simulink model "calibration"  (R2020b)
settings: Solver=VariableStepAuto  StartTime=0.0  StopTime=30  RelTol=1e-3
values from neighbouring files (symbols this model uses):
  aubr = -8:0.05:5    [generate_calibration.m]
  tablebr = zeros(length(vubr),length(aubr))    [generate_calibration.m]
  vubr = 0:0.05:50    [generate_calibration.m]
  x = x-0.1    (= -0.1)    [brake_calibration.m]    (also in thr_calibration.m = 0.05)
libraries: Solver_SF x1
settings Model: Creator=wwcong  LastModifiedBy=mepupu
settings DataIOCC: ReturnWorkspaceOutputs=off
settings DebuggingCC: ArithmeticOperatorsInVariantConditions=warning
settings SFSimCC: SimUseLocalCustomCode=off  CustomCodeUndefinedFunction=UseInterfaceOnly
settings RTWCC: RTWUseLocalCustomCode=off

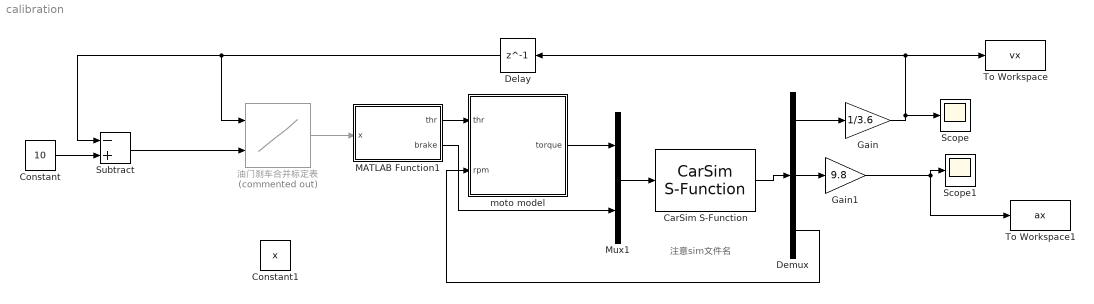
== system calibration ==
  note: 注意sim文件名
  CarSim S-Function : Solver_SF/CarSim S-Function  Priority=1  SIMFILE=simfile.sim
  Constant : Constant  Value=10
  Constant1 : Constant  Value=x
  Delay : Delay  DelayLength=1
  Demux : Demux  Outputs=3
  Gain : Gain  Gain=1/3.6
  Gain1 : Gain  Gain=9.8
  MATLAB Function1 : MATLAB Function  TreatAsAtomicUnit=on
  Mux1 : Mux  Inputs=2
  Scope : Scope
  Scope1 : Scope
  Subtract : Sum  Inputs=-+
  To Workspace : ToWorkspace  VariableName=vx  SaveFormat=Timeseries  SampleTime=0.1
  To Workspace1 : ToWorkspace  VariableName=ax  SaveFormat=Timeseries  SampleTime=0.1
  moto model : MATLAB Function  TreatAsAtomicUnit=on
  油门刹车合并标定表 : Lookup_n-D  Commented=on  BreakpointsForDimension1=vubr  BreakpointsForDimension2=aubr  Table=tablebr  InternalRulePriority=Speed  RndMeth=Simplest  InputSameDT=on
      settings: InputPortMap=u0,u1
  wires:
  CarSim S-Function/1 -> Demux/1
  Demux/1 -> Gain/1
  Demux/2 -> Gain1/1
  Gain1/1 -> To Workspace1/1, Scope1/1
  Gain/1 -> To Workspace/1, Delay/1, Scope/1
  Mux1/1 -> CarSim S-Function/1
  Constant/1 -> Subtract/2
  moto model/1(torque) -> Mux1/1
  MATLAB Function1/1(thr) -> moto model/1(thr)
  MATLAB Function1/2(brake) -> Mux1/2
  Demux/3 -> moto model/2(rpm)
  Subtract/1 -> 油门刹车合并标定表/2
  Delay/1 -> Subtract/1, 油门刹车合并标定表/1
  油门刹车合并标定表/1 -> MATLAB Function1/1(x)

== matlab function calibration/moto model ==
  data: thr input; torque output; rpm input
function torque = fcn(thr,rpm)
Tmax=380*thr;
    if (rpm<=4523)
        torque=Tmax;
    else
        torque=Tmax*4523/rpm;
    end
end

== matlab function calibration/MATLAB Function1 ==
  data: x input; thr output; brake output
function [thr,brake] = fcn(x)
    %正数代表油门，负数代表刹车
    %不允许同时踩油门和刹车
    if x>=0
        thr=x;
        brake=0;
    else
        thr=0;
        brake=-x;
    end
